simulink model "One_Phase_Thyristor_Rectifier"  (R2018b)
settings: Solver=VariableStepAuto  StartTime=0.0  StopTime=10  RelTol=1e-3
libraries: powerlib x9
settings Model: Creator=nailt  LastModifiedBy=fkara
settings DebuggingCC: LibraryContextMissingDiagnostic=none
settings SFSimCC: SimUseLocalCustomCode=off
settings RTWCC: RTWUseLocalCustomCode=off

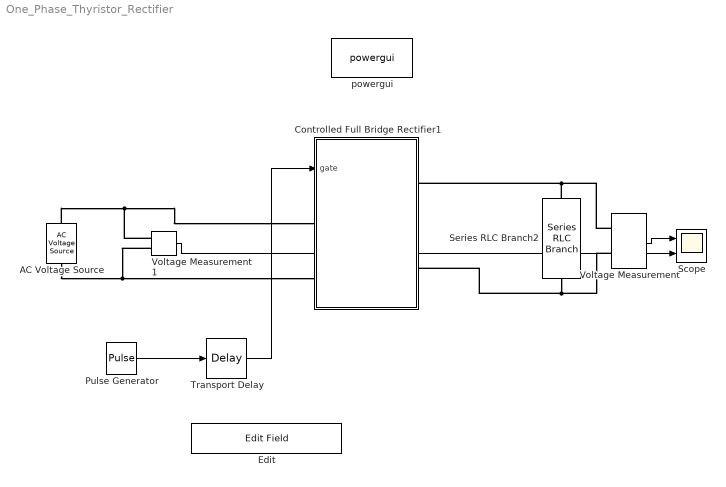
== system One_Phase_Thyristor_Rectifier ==
  AC Voltage Source : powerlib/Electrical Sources/AC Voltage Source  Amplitude=230*sqrt(2)  Phase=0  Frequency=50  SampleTime=0  Measurements=None  BusType=swing  Pref=10e3  Qref=0  Qmin=-inf  Qmax=+inf
      settings: SourceProductName=Simscape Electrical
  Controlled Full Bridge Rectifier1 : Subsystem  AncestorBlock=halfcontrolled/Controlled Full Bridge Rectifier
  Edit : EditField  WebBlockId=182  LabelPosition=Hide  Alignment=Center
  Pulse Generator : DiscretePulseGenerator  PulseType=Time based  Period=0.02  PulseWidth=10
  Scope : Scope  NumInputPorts=2
  Series RLC Branch2 : powerlib/Elements/Series RLC Branch  LConnTagsString=__new0  RConnTagsString=__new0  BranchType=RL  Resistance=4  Inductance=200e-4  SetiL0=off  InitialCurrent=0  Capacitance=1e-6  Setx0=off  InitialVoltage=0  Measurements=None
      settings: SourceProductName=Simscape Electrical
  Transport Delay : TransportDelay  DelayTime=0.02*37.53/360
  Voltage Measurement : powerlib/Measurements/Voltage Measurement  PhasorSimulation=off  OutputType=Complex  PSBequivalent=0
      settings: SourceProductName=Simscape Electrical
  Voltage Measurement1 : powerlib/Measurements/Voltage Measurement  PhasorSimulation=off  OutputType=Complex  PSBequivalent=0
      settings: SourceProductName=Simscape Electrical
  powergui : powerlib/powergui  Priority=1  SimulationMode=Discrete  SampleTime=50e-7  frequency=60  Iterations=50  frequencyindice=0  Pbase=100e6  ErrMax=1e-4  UnitsV=kV  UnitsW=MW  buscounter=0  FunctionMessages=off  echomessages=off  EnableUseOfTLC=off  CurrentSourceSwitches=off  DisableSnubberDevices=off  DisableRonSwitches=off  DisableVfSwitches=off  DisplayEquations=off  SolverType=Tustin/Backward Euler (TBE)  Interpol=off  ExternalGateDelay=off  methode=off  Ts=100  x0status=blocks  SPID=off  SwTol=0  HookPort=off  RestoreLinks=warning  ResistiveCurrentMeasurement=off  Frange=[0:2:500]  Ylog=off  Xlog=on  ShowGrid=off  save=off  variable=ZData  structure=simout  ZoomFFT=off  StartTime=0.0  cycles=3  DisplayStyle=1  fundamental=50  FreqAxis=off  MaxFrequency=1000  frequencyindicesteady=1  RmsSteady=1  display=off
      settings: SourceProductName=Simscape Electrical
  wires:
  Pulse Generator/1 -> Transport Delay/1
  Transport Delay/1 -> Controlled Full Bridge Rectifier1/1(gate)
  Voltage Measurement/1 -> Scope/1
  Voltage Measurement1/1 -> Scope/2
  connections:
  AC Voltage Source/LConn1 -- Voltage Measurement1/LConn2 -- Controlled Full Bridge Rectifier1/LConn2
  AC Voltage Source/RConn1 -- Voltage Measurement1/LConn1 -- Controlled Full Bridge Rectifier1/LConn1
  Series RLC Branch2/RConn1 -- Voltage Measurement/LConn2 -- Controlled Full Bridge Rectifier1/RConn2
  Series RLC Branch2/LConn1 -- Voltage Measurement/LConn1 -- Controlled Full Bridge Rectifier1/RConn1

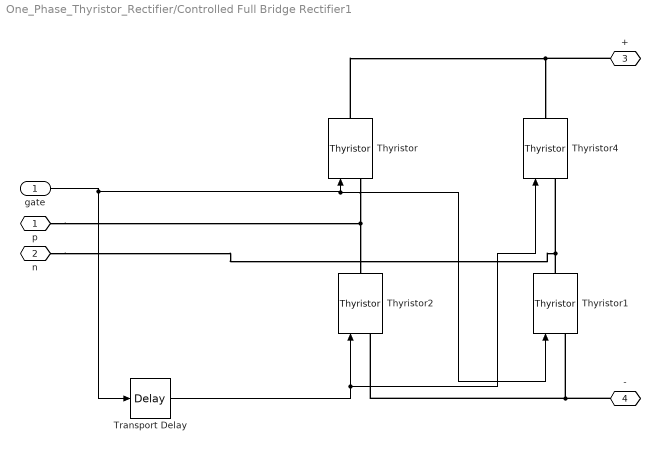
== system One_Phase_Thyristor_Rectifier/Controlled Full Bridge Rectifier1 ==
  gate : Inport
  Thyristor{,1..2,4} (4 alike) : powerlib/Power Electronics/Thyristor  Ron=0.00001  Lon=0  Vf=0  IC=0  Rs=10e9  Cs=250e-12  Measurements=off
      settings: SourceProductName=Simscape Electrical
  Transport Delay : TransportDelay  DelayTime=0.01
  p : PMIOPort  Side=Left
  n : PMIOPort  Port=2  Side=Left
  + : PMIOPort  Port=3  Side=Right
  - : PMIOPort  Port=4  Side=Right
  wires:
  gate/1 -> Thyristor1/1, Thyristor/1, Transport Delay/1
  Transport Delay/1 -> Thyristor4/1, Thyristor2/1
  connections:
  -/RConn1 -- Thyristor2/LConn1 -- Thyristor1/LConn1
  Thyristor1/RConn1 -- n/RConn1 -- Thyristor4/LConn1
  Thyristor/LConn1 -- p/RConn1 -- Thyristor2/RConn1
  +/RConn1 -- Thyristor/RConn1 -- Thyristor4/RConn1
